simulink model "sprezyna"  (R2018b)
settings: Solver=ode4  StartTime=0.0  StopTime=10.0  FixedStep=0.01  RelTol=1e-3
settings Model: Creator=student  LastModifiedBy=student

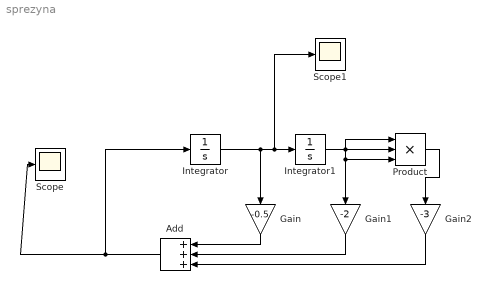
== system sprezyna ==
  Add : Sum  Inputs=+++
  Gain : Gain  Gain=-0.5
  Gain1 : Gain  Gain=-2
  Gain2 : Gain  Gain=-3
  Integrator : Integrator  InitialCondition=1
  Integrator1 : Integrator  InitialCondition=1
  Product : Product  Inputs=3
  Scope : Scope
  Scope1 : Scope
  wires:
  Integrator/1 -> Gain/1, Scope1/1, Integrator1/1
  Gain/1 -> Add/1
  Gain1/1 -> Add/2
  Gain2/1 -> Add/3
  Add/1 -> Integrator/1, Scope/1
  Integrator1/1 -> Product/2, Product/3, Gain1/1, Product/1
  Product/1 -> Gain2/1
